simulink model "GNC_verification"  (R2023a)
settings: Solver=ode4  StartTime=0.0  StopTime=50  FixedStep=0.001  RelTol=1e-3
undefined symbols (not defined in the file): param
libraries: simulink_extras x6, SignalEditorBlockLib x1
settings Model: Creator=timme  LastModifiedBy=timme
settings OptimizationCC: DefaultParameterBehavior=Inlined  UseDivisionForNetSlopeComputation=on  GainParamInheritBuiltInType=on  UseFloatMulNetSlope=on  InlineInvariantSignals=on  EnhancedBackFolding=on  BooleansAsBitfields=on  PassReuseOutputArgsAs=Individual arguments  StateBitsets=on  DataBitsets=on  ZeroExternalMemoryAtStartup=off  ZeroInternalMemoryAtStartup=off  NoFixptDivByZeroProtection=on  EfficientFloat2IntCast=on  LifeSpan=1  OptimizeBlockOrder=speed  DifferentSizesBufferReuse=on  EfficientTunableParamExpr=on
settings DebuggingCC: SignalInfNanChecking=warning  ParameterTunabilityLossMsg=error  AssertControl=DisableAll  VariantConditionMismatch=error
settings HardwareCC: ProdLongLongMode=on
settings SFSimCC: CompileTimeRecursionLimit=0  EnableRuntimeRecursion=off  MATLABDynamicMemAlloc=off
settings RTWCC: Description=Embedded Coder  SystemTargetFile=ert.tlc  TemplateMakefile=ert_default_tmf  TargetLang=C++
settings CodeAppCC: ForceParamTrailComments=on  IgnoreCustomStorageClasses=off  OperatorAnnotations=on  SimulinkDataObjDesc=on  SFDataObjDesc=on  MATLABFcnDesc=on  CustomSymbolStrGlobalVar=rt$N$M  CustomSymbolStrType=$N$M  CustomSymbolStrFcn=$N$M$F  CustomSymbolStrMacro=$N$M  InsertBlockDesc=on
settings ERTTargetCC: TargetLangStandard=C++11 (ISO)  UtilityFuncGeneration=Shared location  GenerateSampleERTMain=on  IncludeMdlTerminateFcn=off  CombineSignalStateStructs=on  CodeInterfacePackaging=C++ class  SupportComplex=off  ParenthesesLevel=Standards  CastingMode=Standards  GenerateSharedConstants=off  InlinedParameterPlacement=NonHierarchical  RootIOFormat=Structure reference  ERTCustomFileTemplate=example_file_process.tlc  ERTFilePackagingFormat=CompactWithDataFile  SuppressUnreachableDefaultCases=off  EnableSignedLeftShifts=off  EnableSignedRightShifts=off

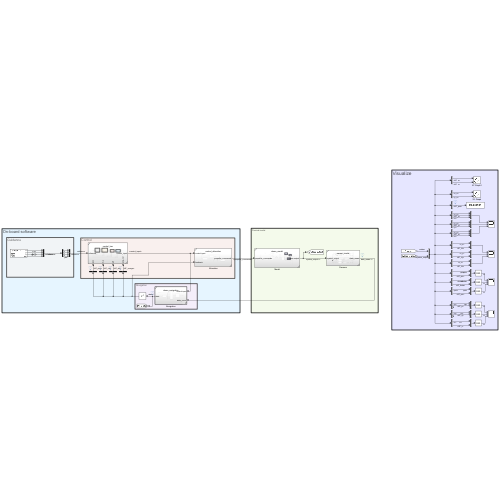
[thumbnail: Simulink's stored preview of the top-level diagram]
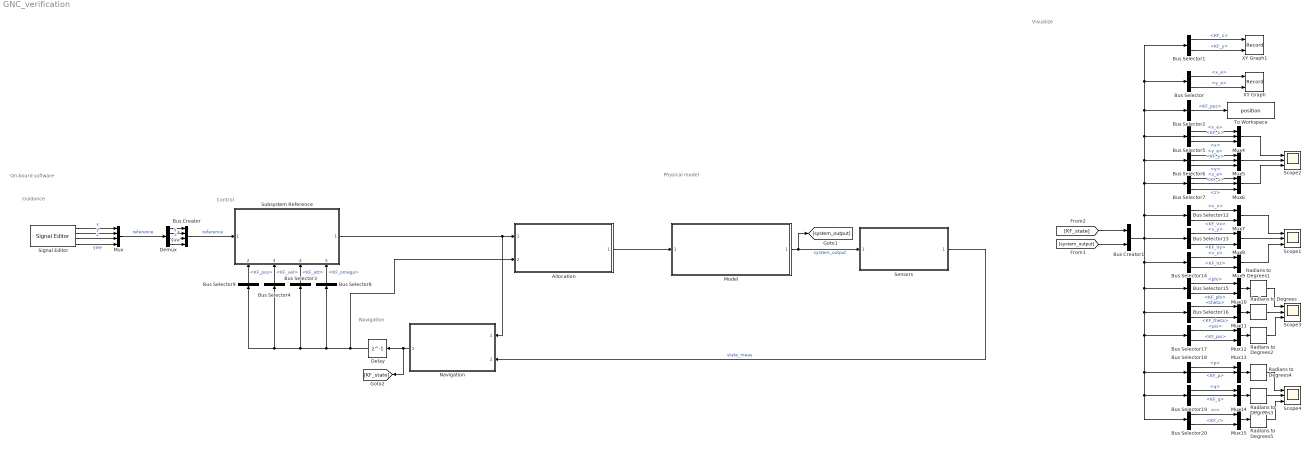
== system GNC_verification ==
  note: Navigation
  note: Control
  note: Physical model
  note: On-board software
  note: Visualize
  note: Guidance
  Allocation : Subsystem  ReferencedSubsystem=control_allocation
  Bus Creator : BusCreator  Inputs=4
  Bus Creator1 : BusCreator  Inputs=2
  Bus Selector : BusSelector  OutputSignals=system_output.pos.x_e,system_output.pos.y_e
  Bus Selector1 : BusSelector  OutputSignals=state.KF_pos.KF_x,state.KF_pos.KF_y
  Bus Selector12 : BusSelector  OutputSignals=system_output.V_e.v_x,state.KF_vel.KF_Vx
  Bus Selector13 : BusSelector  OutputSignals=system_output.V_e.v_y,state.KF_vel.KF_Vy
  Bus Selector14 : BusSelector  OutputSignals=system_output.V_e.v_z,state.KF_vel.KF_Vz
  Bus Selector15 : BusSelector  OutputSignals=system_output.Att.phi,state.KF_att.KF_phi
  Bus Selector16 : BusSelector  OutputSignals=system_output.Att.theta,state.KF_att.KF_theta
  Bus Selector17 : BusSelector  OutputSignals=system_output.Att.psi,state.KF_att.KF_psi
  Bus Selector18 : BusSelector  OutputSignals=system_output.ang_vel.p,state.KF_omega.KF_p,omega_ref.p_ref
  Bus Selector19 : BusSelector  OutputSignals=system_output.ang_vel.q,state.KF_omega.KF_q,omega_ref.q_ref
  Bus Selector2 : BusSelector  OutputSignals=state.KF_pos
  Bus Selector20 : BusSelector  OutputSignals=system_output.ang_vel.r,state.KF_omega.KF_r
  Bus Selector3 : BusSelector  OutputSignals=KF_att
  Bus Selector4 : BusSelector  OutputSignals=KF_vel
  Bus Selector5 : BusSelector  OutputSignals=system_output.pos.x_e,state.KF_pos.KF_x,pos_ref.x
  Bus Selector6 : BusSelector  OutputSignals=system_output.pos.y_e,state.KF_pos.KF_y,pos_ref.y
  Bus Selector7 : BusSelector  OutputSignals=system_output.pos.z_e,state.KF_pos.KF_z,pos_ref.z
  Bus Selector8 : BusSelector  OutputSignals=KF_omega
  Bus Selector9 : BusSelector  OutputSignals=KF_pos
  Delay : Delay  DelayLength=1
  Demux : Demux
  Model : Subsystem  ReferencedSubsystem=drone_model
  Mux : Mux
  Mux{7..12,15} (7 alike) : Mux  Inputs=2
  Mux{4..6,13..14} (5 alike) : Mux  Inputs=3
  Navigation : Subsystem  Description=Navigation module used to estimated the system's state  TreatAsAtomicUnit=on  ReferencedSubsystem=drone_navigation
  Radians to Degrees{,1..5} (6 alike) : simulink_extras/Transformations/Radians to Degrees
  Scope{1..4} (4 alike) : Scope  NumInputPorts=3
  Sensors : Subsystem  ReferencedSubsystem=sensor_model
  Signal Editor : SignalEditorBlockLib/Signal Editor  FileName=full_system_reference.mat  ActiveScenario=verification  ActiveSignal=x  IsBus=off  OutputBusObjectStr=Bus: BusObject  SampleTime=param.dt  ZeroCross=off  OutputAfterFinalValue=Setting to zero  Unit=m  PreserveSignalName=on  ApplySigPropsToAllScenarios=on
  Subsystem Reference : Subsystem  ReferencedSubsystem=control_law
      settings: PortSchema="{\"entries\":[{\"content\":{\"sides\":[{\"content\":{\"connectorIds\":[\"In1\"]},\"type\":\"ConnectorPlacement.EquallySpacedRectSide\",\"uuid\":\"2cee2df0-3d3a-4a29-b454-23d9d03f458c\"},{\"content\":{\"connectorIds\":[\"Out1\"],\"side\":\"RIGHT\"},\"type\":\"ConnectorPlacement.EquallySpacedRectSide\",\"uuid\":\"5651b2ae-0e6e-4567-8068-a5e5b799f50c\"},{\"content\":{\"side\":\"TOP\"},\"type\":\"ConnectorPlacement.EquallySpacedRectSide\",\"uuid\":\"e6d45042-b188-4084-a8d6-3ba5a446321a\"},{\"content\":{\"connectorIds\":[\"In2\",\"In3\",\"In4\",\"In5\"],\"side\":\"BOTTOM\"},\"type\":\"ConnectorPlacement.EquallySpacedRectSide\",\"uuid\":\"fedab0c1-c3ea-4993-b330-4919b97814bf\"}]},\"type\":\"ConnectorPlacement.EquallySpacedConnector\",\"uuid\":\"65e085fb-ac7e-4f5a-a5c0-95474056ab7b\"}],\"packageUris\":[\"http://schema.mathworks.com/mf0/Connector/R2020b\"],\"version\":\"1.0\"}"
  To Workspace : ToWorkspace  VariableName=position  SaveFormat=Timeseries  SampleTime=param.dt
  XY Graph : Record  FileSettingsInternal="{\"entries\":[{\"content\":{\"excelSettings\":{\"content\":{},\"type\":\"Streamout.ExcelSettings\"}},\"type\":\"Streamout.FileSettingStorage\",\"uuid\":\"96c38418-0fbb-476c-bec6-2e95ed6bc886\"}],\"packageUris\":[\"http://schema.mathworks.com/mf0/streamout_blocks/R2020a\"],\"version\":\"1.0\"}"  Layout=[1 1]  SignalsInternal="{\"entries\":[{\"content\":{},\"type\":\"RecordBlkView.InputSignals\",\"uuid\":\"661cee47-8d68-46c9-911c-8b98bf8dafca\"}],\"packageUris\":[\"http://schema.mathworks.com/mf0/streamout_blocks/R2020a\"],\"version\":\"1.0\"}"  VisualizationBindings="{\"xyplotplugin\":{\"info\":[{\"series\":[],\"subplotID\":1}]}}"  CompatibilityTag=XY
  XY Graph1 : Record  FileSettingsInternal="{\"entries\":[{\"content\":{\"excelSettings\":{\"content\":{},\"type\":\"Streamout.ExcelSettings\"}},\"type\":\"Streamout.FileSettingStorage\",\"uuid\":\"03d4d453-e1d1-46f2-a4cb-e1d511c84d8c\"}],\"packageUris\":[\"http://schema.mathworks.com/mf0/streamout_blocks/R2020a\"],\"version\":\"1.0\"}"  Layout=[1 1]  SignalsInternal="{\"entries\":[{\"content\":{},\"type\":\"RecordBlkView.InputSignals\",\"uuid\":\"c0f91c0c-945a-4aeb-a3b9-9664774de9ce\"}],\"packageUris\":[\"http://schema.mathworks.com/mf0/streamout_blocks/R2020a\"],\"version\":\"1.0\"}"  VisualizationBindings="{\"xyplotplugin\":{\"info\":[{\"series\":[],\"subplotID\":1}]}}"  CompatibilityTag=XY
  wires:
  Bus Selector5/1 -> Mux4/1  "<x_e>"
  Bus Selector5/2 -> Mux4/2  "<KF_x>"
  Bus Selector6/1 -> Mux5/1  "<y_e>"
  Bus Selector6/2 -> Mux5/2  "<KF_y>"
  Bus Selector7/2 -> Mux6/2  "<KF_z>"
  Bus Selector7/1 -> Mux6/1  "<z_e>"
  Bus Selector12/2 -> Mux7/2  "<KF_Vx>"
  Bus Selector12/1 -> Mux7/1  "<v_x>"
  Bus Selector13/1 -> Mux8/1  "<v_y>"
  Bus Selector14/2 -> Mux9/2  "<KF_Vz>"
  Bus Selector14/1 -> Mux9/1  "<v_z>"
  Bus Selector13/2 -> Mux8/2  "<KF_Vy>"
  Bus Selector16/2 -> Mux11/2  "<KF_theta>"
  Mux12/1 -> Radians to Degrees2/1
  Mux11/1 -> Radians to Degrees/1
  Bus Selector17/2 -> Mux12/2  "<KF_psi>"
  Bus Selector15/2 -> Mux10/2  "<KF_phi>"
  Mux10/1 -> Radians to Degrees1/1
  Bus Selector19/2 -> Mux14/2  "<KF_q>"
  Bus Selector18/2 -> Mux13/2  "<KF_p>"
  Mux13/1 -> Radians to Degrees4/1
  Bus Selector20/1 -> Mux15/1  "<r>"
  Bus Selector18/1 -> Mux13/1  "<p>"
  Mux15/1 -> Radians to Degrees5/1
  Bus Selector20/2 -> Mux15/2  "<KF_r>"
  Mux14/1 -> Radians to Degrees3/1
  Bus Selector19/1 -> Mux14/1  "<q>"
  Bus Selector/1 -> XY Graph/1  "<x_e>"
  Bus Selector/2 -> XY Graph/2  "<y_e>"
  Mux5/1 -> Scope2/2
  Mux4/1 -> Scope2/1
  Mux6/1 -> Scope2/3
  Mux8/1 -> Scope1/2
  Mux9/1 -> Scope1/3
  Mux7/1 -> Scope1/1
  Radians to Degrees2/1 -> Scope3/3
  Radians to Degrees1/1 -> Scope3/1
  Radians to Degrees/1 -> Scope3/2
  Radians to Degrees5/1 -> Scope4/3
  Radians to Degrees4/1 -> Scope4/1
  Radians to Degrees3/1 -> Scope4/2
  Bus Selector1/1 -> XY Graph1/1  "<KF_x>"
  Bus Selector1/2 -> XY Graph1/2  "<KF_y>"
  Navigation/1 -> [KF_state], Delay/1
  Bus Selector2/1 -> To Workspace/1  "<KF_pos>"
  Bus Creator1/1 -> Bus Selector12/1, Bus Selector7/1, Bus Selector6/1, Bus Selector2/1, Bus Selector1/1, Bus Selector/1, Bus Selector5/1, Bus Selector14/1, Bus Selector20/1, Bus Selector19/1, Bus Selector18/1, Bus Selector17/1, Bus Selector16/1, Bus Selector15/1, Bus Selector13/1
  Bus Selector8/1 -> Subsystem Reference/5  "<KF_omega>"
  Sensors/1 -> Navigation/2  "state_meas"
  Model/1 -> Sensors/1, [system_output]  "system_output"
  [system_output] -> Bus Creator1/2
  [KF_state] -> Bus Creator1/1
  Bus Selector3/1 -> Subsystem Reference/4  "<KF_att>"
  Bus Selector15/1 -> Mux10/1  "<phi>"
  Bus Selector16/1 -> Mux11/1  "<theta>"
  Bus Selector17/1 -> Mux12/1  "<psi>"
  Bus Selector4/1 -> Subsystem Reference/3  "<KF_vel>"
  Bus Selector9/1 -> Subsystem Reference/2  "<KF_pos>"
  Bus Selector5/3 -> Mux4/3  "<x>"
  Bus Selector6/3 -> Mux5/3  "<y>"
  Bus Selector7/3 -> Mux6/3  "<z>"
  Subsystem Reference/1 -> Navigation/1, Allocation/1
  Allocation/1 -> Model/1
  Delay/1 -> Bus Selector9/1, Bus Selector4/1, Bus Selector3/1, Bus Selector8/1, Allocation/2
  Signal Editor/2 -> Mux/2  "y"
  Signal Editor/4 -> Mux/4  "yaw"
  Signal Editor/3 -> Mux/3  "z"
  Demux/1 -> Bus Creator/1  "x"
  Demux/4 -> Bus Creator/4  "yaw"
  Mux/1 -> Demux/1  "reference"
  Bus Creator/1 -> Subsystem Reference/1  "reference"
  Demux/2 -> Bus Creator/2  "y"
  Demux/3 -> Bus Creator/3  "z"
  Signal Editor/1 -> Mux/1  "x"
